simulink model "VSCHVDCunitblackstart"  (R2025b)
settings: Solver=VariableStepAuto  StartTime=0  StopTime=25  FixedStep=5e-5  RelTol=1e-3
PreLoadFcn:
  | HVDCParameters;
  | BlackStartMMCParameters;
undefined symbols (not defined in the file): DiscIntNeverNeededParam, FRated, frt, gGFM, grid, Lbase, Lr, Lt, lvrt, mGFM, mpptOmega, mpptWindSpeed, Nm, pmsm, PRated, Rc, rpir, Rr, Rt, time, Tpir, Ts, Vbase, Vdcs0, VRated, Vt2, windController, windTurbine, Zbase
libraries: fl_lib x47, ee_lib x41, nesl_utility x33, eeGeneralControl x13, eeTransforms x12, slpidlib x8, eeSinusoidalMeasurementV2 x4, simulink x2, eeSinusoidalMeasurement x1, eeStairGenerator x1
(part 2 of 5)

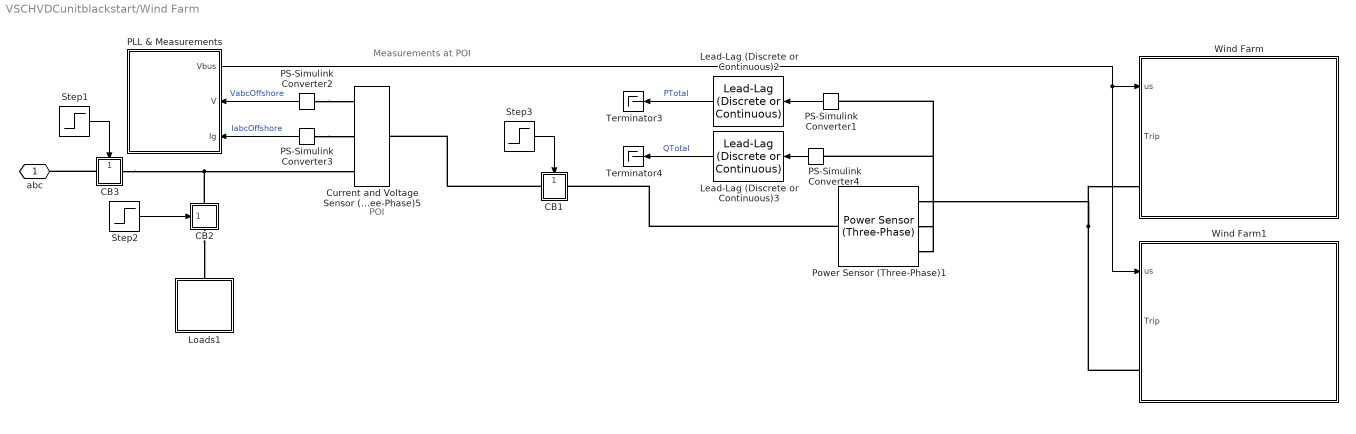
== system VSCHVDCunitblackstart/Wind Farm ==
  note: POI
  note: Measurements at POI
  CB1 : Subsystem
      settings: PortSchema="{\"entries\":[{\"content\":{\"sides\":[{\"content\":{\"connectorIds\":[\"LConn1\"]},\"type\":\"ConnectorPlacement.EquallySpacedRectSide\",\"uuid\":\"67c0f727-7c15-41c9-98df-b3c7d57498ed\"},{\"content\":{\"connectorIds\":[\"RConn1\"],\"side\":\"RIGHT\"},\"type\":\"ConnectorPlacement.EquallySpacedRectSide\",\"uuid\":\"7fc39429-ba61-416d-b42b-93e81eb2f426\"},{\"content\":{\"side\":\"TOP\"},\"type\":\"ConnectorPlacement.EquallySpacedRectSide\",\"uuid\":\"c6dd9263-b57a-4cff-a218-af99f2798f29\"},{\"content\":{\"connectorIds\":[\"In1\"],\"side\":\"BOTTOM\"},\"type\":\"ConnectorPlacement.EquallySpacedRectSide\",\"uuid\":\"e2a2ba44-d59d-4e27-adf1-3f94e828ca78\"}]},\"type\":\"ConnectorPlacement.EquallySpacedConnector\",\"uuid\":\"b349a99b-c902-4df9-9c99-34841afb28dd\"}],\"packageUris\":[\"http://schema.mathworks.com/mf0/Connector/R2020b\"],\"version\":\"1.0\"}"
  CB2 : Subsystem
      settings: PortSchema="{\"entries\":[{\"content\":{\"sides\":[{\"content\":{\"connectorIds\":[\"LConn1\"]},\"type\":\"ConnectorPlacement.EquallySpacedRectSide\",\"uuid\":\"67c0f727-7c15-41c9-98df-b3c7d57498ed\"},{\"content\":{\"connectorIds\":[\"RConn1\"],\"side\":\"RIGHT\"},\"type\":\"ConnectorPlacement.EquallySpacedRectSide\",\"uuid\":\"7fc39429-ba61-416d-b42b-93e81eb2f426\"},{\"content\":{\"side\":\"TOP\"},\"type\":\"ConnectorPlacement.EquallySpacedRectSide\",\"uuid\":\"c6dd9263-b57a-4cff-a218-af99f2798f29\"},{\"content\":{\"connectorIds\":[\"In1\"],\"side\":\"BOTTOM\"},\"type\":\"ConnectorPlacement.EquallySpacedRectSide\",\"uuid\":\"e2a2ba44-d59d-4e27-adf1-3f94e828ca78\"}]},\"type\":\"ConnectorPlacement.EquallySpacedConnector\",\"uuid\":\"b349a99b-c902-4df9-9c99-34841afb28dd\"}],\"packageUris\":[\"http://schema.mathworks.com/mf0/Connector/R2020b\"],\"version\":\"1.0\"}"
  CB3 : Subsystem
      settings: PortSchema="{\"entries\":[{\"content\":{\"sides\":[{\"content\":{\"connectorIds\":[\"LConn1\"]},\"type\":\"ConnectorPlacement.EquallySpacedRectSide\",\"uuid\":\"67c0f727-7c15-41c9-98df-b3c7d57498ed\"},{\"content\":{\"connectorIds\":[\"RConn1\"],\"side\":\"RIGHT\"},\"type\":\"ConnectorPlacement.EquallySpacedRectSide\",\"uuid\":\"7fc39429-ba61-416d-b42b-93e81eb2f426\"},{\"content\":{\"side\":\"TOP\"},\"type\":\"ConnectorPlacement.EquallySpacedRectSide\",\"uuid\":\"c6dd9263-b57a-4cff-a218-af99f2798f29\"},{\"content\":{\"connectorIds\":[\"In1\"],\"side\":\"BOTTOM\"},\"type\":\"ConnectorPlacement.EquallySpacedRectSide\",\"uuid\":\"e2a2ba44-d59d-4e27-adf1-3f94e828ca78\"}]},\"type\":\"ConnectorPlacement.EquallySpacedConnector\",\"uuid\":\"b349a99b-c902-4df9-9c99-34841afb28dd\"}],\"packageUris\":[\"http://schema.mathworks.com/mf0/Connector/R2020b\"],\"version\":\"1.0\"}"
  Current and Voltage Sensor (Three-Phase)5 : ee_lib/Sensors & Transducers/Current and Voltage Sensor (Three-Phase)  vMeasurementType=ee.enum.vmeasurement.lg  outputUnit=ee.enum.unit.pu  SRated=base.mVA A*V  VRated=base.kV V  I_specify=off  I_priority=None  I=[0, 0, 0] A  I_nominal_specify=off  I_nominal_value=1  I_nominal_unit=A  V_specify=off  V_priority=None  V=[0, 0, 0] V  V_nominal_specify=off  V_nominal_value=1  V_nominal_unit=V
      settings: InternalSimscapePortConfiguration="{\"Bottom\":[],\"Left\":[{\"id\":\"N1\",\"label\":\"~1\",\"type\":\"foundation.electrical.three_phase\"}],\"Right\":[{\"id\":\"V_output\",\"label\":\"V\",\"type\":\"output\"},{\"id\":\"I_output\",\"label\":\"I\",\"type\":\"output\"},{\"id\":\"N2\",\"label\":\"~2\",\"type\":\"foundation.electrical.three_phase\"}],\"Top\":[]}"
  Lead-Lag (Discrete or Continuous)2 : eeGeneralControl/Lead-Lag (Discrete or Continuous)  T1=0  T2=windController.tSensor  B=inf  A=-inf  init_option=Inherited from block input  x0=0  Ts=Ts
      settings: LibrarySourceBlock=|
      | ee_sl_lib/General Control/Lead-Lag
      | (Discrete or Continuous)
  Lead-Lag (Discrete or Continuous)3 : eeGeneralControl/Lead-Lag (Discrete or Continuous)  T1=0  T2=windController.tSensor  B=inf  A=-inf  init_option=Inherited from block input  x0=0  Ts=Ts
      settings: LibrarySourceBlock=|
      | ee_sl_lib/General Control/Lead-Lag
      | (Discrete or Continuous)
  Loads1 : Subsystem
      mask Display: image('Load_2.png');
  PLL & Measurements : Subsystem
      settings: PortSchema="{\"entries\":[{\"content\":{\"sides\":[{\"content\":{\"connectorIds\":[\"Out1\",\"In1\",\"In2\"]},\"type\":\"ConnectorPlacement.EquallySpacedRectSide\",\"uuid\":\"76485780-20fe-4fcf-8224-69648da6ed2a\"},{\"content\":{\"side\":\"RIGHT\"},\"type\":\"ConnectorPlacement.EquallySpacedRectSide\",\"uuid\":\"f19a6390-e634-42c7-8d46-4cd80cbab182\"},{\"content\":{\"side\":\"TOP\"},\"type\":\"ConnectorPlacement.EquallySpacedRectSide\",\"uuid\":\"87682f72-1844-428e-be70-ad7ca3191ee3\"}]},\"type\":\"ConnectorPlacement.EquallySpacedConnector\",\"uuid\":\"f2136b07-48ec-402b-adb3-18c0bac2157c\"}],\"packageUris\":[\"http://schema.mathworks.com/mf0/Connector/R2020b\"],\"version\":\"1.0\"}"
      mask Display: image('measurements.png'); % Use "Edit Image" on toolstrip to change.
  PS-Simulink Converter{1..4} (4 alike) : nesl_utility/PS-Simulink Converter  PhysicalDomain=network_engine_domain  SubClassName=ps_output  LeftPortType=input  RightPortType=output  PseudoPeriodic=off  Frequencies=[]  VectorFormat=inherit  Unit=inherit  AffineConversion=off
  Power Sensor (Three-Phase)1 : ee_lib/Sensors & Transducers/Power Sensor (Three-Phase)  load_type=ee.enum.passive.type_balanced.balanced  f0=60 Hz
      settings: InternalSimscapePortConfiguration="{\"Bottom\":[],\"Left\":[{\"id\":\"N1\",\"label\":\"~1\",\"type\":\"foundation.electrical.three_phase\"}],\"Right\":[{\"id\":\"N2\",\"label\":\"~2\",\"type\":\"foundation.electrical.three_phase\"}],\"Top\":[{\"id\":\"Pm\",\"label\":\"P\",\"type\":\"output\"},{\"id\":\"Qm\",\"label\":\"Q\",\"type\":\"output\"}]}"
  Step1 : Step  Time=9  Before=1  After=0  SampleTime=Ts
  Step2 : Step  Time=3  Before=1  After=0  SampleTime=Ts
  Step3 : Step  Time=2  Before=1  After=0  SampleTime=Ts
  Terminator3 : Terminator
  Terminator4 : Terminator
  Wind Farm : Subsystem
      settings: PortSchema="{\"entries\":[{\"content\":{\"sides\":[{\"content\":{\"connectorIds\":[\"In1\",\"Out1\",\"LConn1\"]},\"type\":\"ConnectorPlacement.EquallySpacedRectSide\",\"uuid\":\"1189e956-e6f0-4ada-905a-6b9abec668a8\"},{\"content\":{\"side\":\"RIGHT\"},\"type\":\"ConnectorPlacement.EquallySpacedRectSide\",\"uuid\":\"3ddb8f28-1c9c-423f-814f-a5e5ca919d79\"},{\"content\":{\"side\":\"TOP\"},\"type\":\"ConnectorPlacement.EquallySpacedRectSide\",\"uuid\":\"c360f229-efd7-488e-97f8-90fd9e6e05d4\"},{\"content\":{\"side\":\"BOTTOM\"},\"type\":\"ConnectorPlacement.EquallySpacedRectSide\",\"uuid\":\"99811ca4-1621-4e62-9767-ce3bd58f839c\"}]},\"type\":\"ConnectorPlacement.EquallySpacedConnector\",\"uuid\":\"16843f42-9f9b-4252-a0c2-a64badb15c83\"}],\"packageUris\":[\"http://schema.mathworks.com/mf0/Connector/R2020b\"],\"version\":\"1.0\"}"
      mask Display: image('WindFarmModel4_1.PNG');
  Wind Farm1 : Subsystem
      settings: PortSchema="{\"entries\":[{\"content\":{\"sides\":[{\"content\":{\"connectorIds\":[\"In1\",\"Out1\",\"LConn1\"]},\"type\":\"ConnectorPlacement.EquallySpacedRectSide\",\"uuid\":\"1189e956-e6f0-4ada-905a-6b9abec668a8\"},{\"content\":{\"side\":\"RIGHT\"},\"type\":\"ConnectorPlacement.EquallySpacedRectSide\",\"uuid\":\"3ddb8f28-1c9c-423f-814f-a5e5ca919d79\"},{\"content\":{\"side\":\"TOP\"},\"type\":\"ConnectorPlacement.EquallySpacedRectSide\",\"uuid\":\"c360f229-efd7-488e-97f8-90fd9e6e05d4\"},{\"content\":{\"side\":\"BOTTOM\"},\"type\":\"ConnectorPlacement.EquallySpacedRectSide\",\"uuid\":\"99811ca4-1621-4e62-9767-ce3bd58f839c\"}]},\"type\":\"ConnectorPlacement.EquallySpacedConnector\",\"uuid\":\"16843f42-9f9b-4252-a0c2-a64badb15c83\"}],\"packageUris\":[\"http://schema.mathworks.com/mf0/Connector/R2020b\"],\"version\":\"1.0\"}"
      mask Display: image('WindFarmModel4_1.PNG');
  abc : PMIOPort  Side=Right
  wires:
  PS-Simulink Converter2/1 -> PLL & Measurements/1(V)  "VabcOffshore"
  PS-Simulink Converter3/1 -> PLL & Measurements/2(Ig)  "IabcOffshore"
  Step3/1 -> CB1/1(input0)
  Step2/1 -> CB2/1(input0)
  PLL & Measurements/1(Vbus) -> Wind Farm1/1(us), Wind Farm/1(us)
  Step1/1 -> CB3/1(input0)
  Lead-Lag (Discrete or Continuous)2/1 -> Terminator3/1  "PTotal"
  PS-Simulink Converter1/1 -> Lead-Lag (Discrete or Continuous)2/1
  PS-Simulink Converter4/1 -> Lead-Lag (Discrete or Continuous)3/1
  Lead-Lag (Discrete or Continuous)3/1 -> Terminator4/1  "QTotal"
  connections:
  CB2/RConn1 -- CB3/RConn1 -- Current and Voltage Sensor (Three-Phase)5/RConn3
  CB2/LConn1 -- Loads1/RConn1
  CB1/LConn1 -- Current and Voltage Sensor (Three-Phase)5/LConn1
  PS-Simulink Converter2/LConn1 -- Current and Voltage Sensor (Three-Phase)5/RConn1
  PS-Simulink Converter3/LConn1 -- Current and Voltage Sensor (Three-Phase)5/RConn2
  Wind Farm1/LConn1 -- Power Sensor (Three-Phase)1/LConn1 -- Wind Farm/LConn1
  CB3/LConn1 -- abc/RConn1
  Power Sensor (Three-Phase)1/LConn3 -- PS-Simulink Converter4/LConn1
  Power Sensor (Three-Phase)1/LConn2 -- PS-Simulink Converter1/LConn1
  Power Sensor (Three-Phase)1/RConn1 -- CB1/RConn1

== system VSCHVDCunitblackstart/Cables/Idcnr ==
  Current Sensor : fl_lib/Electrical/Electrical Sensors/Current Sensor
  PS-Simulink Converter : nesl_utility/PS-Simulink Converter  PhysicalDomain=network_engine_domain  SubClassName=ps_output  LeftPortType=input  RightPortType=output  PseudoPeriodic=off  Frequencies=[]  VectorFormat=1-D array  Unit=A  AffineConversion=off
  + : PMIOPort  Side=Left
  - : PMIOPort  Port=2  Side=Right
  i : Outport
  wires:
  PS-Simulink Converter/1 -> i/1
  connections:
  -/RConn1 -- Current Sensor/RConn2
  Current Sensor/LConn1 -- +/RConn1
  PS-Simulink Converter/LConn1 -- Current Sensor/RConn1

== system VSCHVDCunitblackstart/Cables/Idcns ==
  Current Sensor : fl_lib/Electrical/Electrical Sensors/Current Sensor
  PS-Simulink Converter : nesl_utility/PS-Simulink Converter  PhysicalDomain=network_engine_domain  SubClassName=ps_output  LeftPortType=input  RightPortType=output  PseudoPeriodic=off  Frequencies=[]  VectorFormat=1-D array  Unit=A  AffineConversion=off
  + : PMIOPort  Side=Left
  - : PMIOPort  Port=2  Side=Right
  i : Outport
  wires:
  PS-Simulink Converter/1 -> i/1
  connections:
  PS-Simulink Converter/LConn1 -- Current Sensor/RConn1
  Current Sensor/LConn1 -- +/RConn1
  -/RConn1 -- Current Sensor/RConn2

== system VSCHVDCunitblackstart/Cables/Idcpr ==
  Current Sensor : fl_lib/Electrical/Electrical Sensors/Current Sensor
  PS-Simulink Converter : nesl_utility/PS-Simulink Converter  PhysicalDomain=network_engine_domain  SubClassName=ps_output  LeftPortType=input  RightPortType=output  PseudoPeriodic=off  Frequencies=[]  VectorFormat=1-D array  Unit=A  AffineConversion=off
  + : PMIOPort  Side=Left
  - : PMIOPort  Port=2  Side=Right
  i : Outport
  wires:
  PS-Simulink Converter/1 -> i/1
  connections:
  PS-Simulink Converter/LConn1 -- Current Sensor/RConn1
  Current Sensor/LConn1 -- +/RConn1
  -/RConn1 -- Current Sensor/RConn2

== system VSCHVDCunitblackstart/Cables/Idcps ==
  Current Sensor : fl_lib/Electrical/Electrical Sensors/Current Sensor
  PS-Simulink Converter : nesl_utility/PS-Simulink Converter  PhysicalDomain=network_engine_domain  SubClassName=ps_output  LeftPortType=input  RightPortType=output  PseudoPeriodic=off  Frequencies=[]  VectorFormat=1-D array  Unit=A  AffineConversion=off
  + : PMIOPort  Side=Left
  - : PMIOPort  Port=2  Side=Right
  i : Outport
  wires:
  PS-Simulink Converter/1 -> i/1
  connections:
  -/RConn1 -- Current Sensor/RConn2
  Current Sensor/LConn1 -- +/RConn1
  PS-Simulink Converter/LConn1 -- Current Sensor/RConn1

== system VSCHVDCunitblackstart/Cables/Vdcnr ==
  PS-Simulink Converter : nesl_utility/PS-Simulink Converter  PhysicalDomain=network_engine_domain  SubClassName=ps_output  LeftPortType=input  RightPortType=output  PseudoPeriodic=off  Frequencies=[]  VectorFormat=1-D array  Unit=V  AffineConversion=off
  Voltage Sensor : fl_lib/Electrical/Electrical Sensors/Voltage Sensor
  + : PMIOPort  Side=Left
  - : PMIOPort  Port=2  Side=Right
  v : Outport
  wires:
  PS-Simulink Converter/1 -> v/1
  connections:
  PS-Simulink Converter/LConn1 -- Voltage Sensor/RConn1
  Voltage Sensor/RConn2 -- -/RConn1
  Voltage Sensor/LConn1 -- +/RConn1

== system VSCHVDCunitblackstart/Cables/Vdcns ==
  PS-Simulink Converter : nesl_utility/PS-Simulink Converter  PhysicalDomain=network_engine_domain  SubClassName=ps_output  LeftPortType=input  RightPortType=output  PseudoPeriodic=off  Frequencies=[]  VectorFormat=1-D array  Unit=V  AffineConversion=off
  Voltage Sensor : fl_lib/Electrical/Electrical Sensors/Voltage Sensor
  + : PMIOPort  Side=Left
  - : PMIOPort  Port=2  Side=Right
  v : Outport
  wires:
  PS-Simulink Converter/1 -> v/1
  connections:
  Voltage Sensor/LConn1 -- +/RConn1
  Voltage Sensor/RConn2 -- -/RConn1
  PS-Simulink Converter/LConn1 -- Voltage Sensor/RConn1

== system VSCHVDCunitblackstart/Cables/Vdcpr ==
  PS-Simulink Converter : nesl_utility/PS-Simulink Converter  PhysicalDomain=network_engine_domain  SubClassName=ps_output  LeftPortType=input  RightPortType=output  PseudoPeriodic=off  Frequencies=[]  VectorFormat=1-D array  Unit=V  AffineConversion=off
  Voltage Sensor : fl_lib/Electrical/Electrical Sensors/Voltage Sensor
  + : PMIOPort  Side=Left
  - : PMIOPort  Port=2  Side=Right
  v : Outport
  wires:
  PS-Simulink Converter/1 -> v/1
  connections:
  Voltage Sensor/LConn1 -- +/RConn1
  Voltage Sensor/RConn2 -- -/RConn1
  PS-Simulink Converter/LConn1 -- Voltage Sensor/RConn1

== system VSCHVDCunitblackstart/Cables/Vdcps ==
  PS-Simulink Converter : nesl_utility/PS-Simulink Converter  PhysicalDomain=network_engine_domain  SubClassName=ps_output  LeftPortType=input  RightPortType=output  PseudoPeriodic=off  Frequencies=[]  VectorFormat=1-D array  Unit=V  AffineConversion=off
  Voltage Sensor : fl_lib/Electrical/Electrical Sensors/Voltage Sensor
  + : PMIOPort  Side=Left
  - : PMIOPort  Port=2  Side=Right
  v : Outport
  wires:
  PS-Simulink Converter/1 -> v/1
  connections:
  PS-Simulink Converter/LConn1 -- Voltage Sensor/RConn1
  Voltage Sensor/RConn2 -- -/RConn1
  Voltage Sensor/LConn1 -- +/RConn1

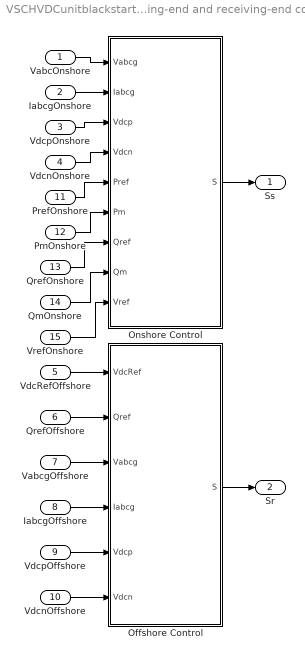
== system VSCHVDCunitblackstart/Control/Sending-end and receiving-end control ==
  VabcOnshore : Inport
  IabcgOnshore : Inport  Port=2
  VdcpOnshore : Inport  Port=3
  VdcnOnshore : Inport  Port=4
  VdcRefOffshore : Inport  Port=5
  QrefOffshore : Inport  Port=6
  VabcgOffshore : Inport  Port=7
  IabcgOffshore : Inport  Port=8
  VdcpOffshore : Inport  Port=9
  VdcnOffshore : Inport  Port=10
  PrefOnshore : Inport  Port=11
  PmOnshore : Inport  Port=12
  QrefOnshore : Inport  Port=13
  QmOnshore : Inport  Port=14
  VrefOnshore : Inport  Port=15
  Offshore Control : Subsystem  VariantControl=ControllerTimeMode
  Onshore Control : Subsystem  VariantControl=ControllerTimeMode
  Ss : Outport
  Sr : Outport  Port=2
  wires:
  QrefOffshore/1 -> Offshore Control/2(Qref)
  VabcgOffshore/1 -> Offshore Control/3(Vabcg)
  VdcnOffshore/1 -> Offshore Control/6(Vdcn)
  VdcpOffshore/1 -> Offshore Control/5(Vdcp)
  VdcnOnshore/1 -> Onshore Control/4(Vdcn)
  VdcRefOffshore/1 -> Offshore Control/1(VdcRef)
  Offshore Control/1(S) -> Sr/1
  IabcgOffshore/1 -> Offshore Control/4(Iabcg)
  IabcgOnshore/1 -> Onshore Control/2(Iabcg)
  VdcpOnshore/1 -> Onshore Control/3(Vdcp)
  VabcOnshore/1 -> Onshore Control/1(Vabcg)
  Onshore Control/1(S) -> Ss/1
  PrefOnshore/1 -> Onshore Control/5(Pref)
  PmOnshore/1 -> Onshore Control/6(Pm)
  QrefOnshore/1 -> Onshore Control/7(Qref)
  QmOnshore/1 -> Onshore Control/8(Qm)
  VrefOnshore/1 -> Onshore Control/9(Vref)

== system VSCHVDCunitblackstart/Offshore Station/Receiving-end vi ==
  Current and Voltage Sensor (Three-Phase) : ee_lib/Sensors & Transducers/Current and Voltage Sensor (Three-Phase)  vMeasurementType=ee.enum.vmeasurement.lg  outputUnit=ee.enum.unit.pu  SRated=PRated W  VRated=VgridRated V  I_specify=off  I_priority=None  I=[0, 0, 0] A  I_nominal_specify=off  I_nominal_value=1  I_nominal_unit=A  V_specify=off  V_priority=None  V=[0, 0, 0] V  V_nominal_specify=off  V_nominal_value=1  V_nominal_unit=V
      settings: InternalSimscapePortConfiguration="{\"Bottom\":[],\"Left\":[{\"id\":\"N1\",\"label\":\"~1\",\"type\":\"foundation.electrical.three_phase\"}],\"Right\":[{\"id\":\"V_output\",\"label\":\"V\",\"type\":\"output\"},{\"id\":\"I_output\",\"label\":\"I\",\"type\":\"output\"},{\"id\":\"N2\",\"label\":\"~2\",\"type\":\"foundation.electrical.three_phase\"}],\"Top\":[]}"
  PS-Simulink Converter : nesl_utility/PS-Simulink Converter  PhysicalDomain=network_engine_domain  SubClassName=ps_output  LeftPortType=input  RightPortType=output  PseudoPeriodic=off  Frequencies=[]  VectorFormat=1-D array  Unit=1  AffineConversion=off
  PS-Simulink Converter2 : nesl_utility/PS-Simulink Converter  PhysicalDomain=network_engine_domain  SubClassName=ps_output  LeftPortType=input  RightPortType=output  PseudoPeriodic=off  Frequencies=[]  VectorFormat=1-D array  Unit=1  AffineConversion=off
  ~1 : PMIOPort  Side=Left
  ~2 : PMIOPort  Port=2  Side=Right
  v : Outport
  i : Outport  Port=2
  wires:
  PS-Simulink Converter/1 -> i/1
  PS-Simulink Converter2/1 -> v/1
  connections:
  Current and Voltage Sensor (Three-Phase)/LConn1 -- ~1/RConn1
  Current and Voltage Sensor (Three-Phase)/RConn2 -- PS-Simulink Converter/LConn1
  PS-Simulink Converter2/LConn1 -- Current and Voltage Sensor (Three-Phase)/RConn1
  ~2/RConn1 -- Current and Voltage Sensor (Three-Phase)/RConn3

== system VSCHVDCunitblackstart/Onshore Grid/CB1 ==
  input0 : Inport
  Subsystem1 : Subsystem
      settings: PortSchema="{\"entries\":[{\"content\":{\"sides\":[{\"content\":{\"connectorIds\":[\"LConn1\",\"In1\"]},\"type\":\"ConnectorPlacement.EquallySpacedRectSide\",\"uuid\":\"4d523b2f-3490-490d-9193-0c3e52b1c3a1\"},{\"content\":{\"connectorIds\":[\"RConn1\"],\"side\":\"RIGHT\"},\"type\":\"ConnectorPlacement.EquallySpacedRectSide\",\"uuid\":\"1543a14a-65b5-4637-8d41-6da95a6ca307\"},{\"content\":{\"side\":\"TOP\"},\"type\":\"ConnectorPlacement.EquallySpacedRectSide\",\"uuid\":\"9fff8ee8-4727-466f-977a-681c4f14cc56\"}]},\"type\":\"ConnectorPlacement.EquallySpacedConnector\",\"uuid\":\"a46df766-bf17-4bd6-a8b3-579011040ee9\"}],\"packageUris\":[\"http://schema.mathworks.com/mf0/Connector/R2020b\"],\"version\":\"1.0\"}"
  Conn2 : PMIOPort  Side=Left
  Conn1 : PMIOPort  Port=2  Side=Right
  wires:
  input0/1 -> Subsystem1/1(input0)
  connections:
  Conn2/RConn1 -- Subsystem1/RConn1
  Subsystem1/LConn1 -- Conn1/RConn1

== system VSCHVDCunitblackstart/Onshore Grid/CB2 ==
  input0 : Inport
  Subsystem1 : Subsystem
      settings: PortSchema="{\"entries\":[{\"content\":{\"sides\":[{\"content\":{\"connectorIds\":[\"LConn1\",\"In1\"]},\"type\":\"ConnectorPlacement.EquallySpacedRectSide\",\"uuid\":\"4d523b2f-3490-490d-9193-0c3e52b1c3a1\"},{\"content\":{\"connectorIds\":[\"RConn1\"],\"side\":\"RIGHT\"},\"type\":\"ConnectorPlacement.EquallySpacedRectSide\",\"uuid\":\"1543a14a-65b5-4637-8d41-6da95a6ca307\"},{\"content\":{\"side\":\"TOP\"},\"type\":\"ConnectorPlacement.EquallySpacedRectSide\",\"uuid\":\"9fff8ee8-4727-466f-977a-681c4f14cc56\"}]},\"type\":\"ConnectorPlacement.EquallySpacedConnector\",\"uuid\":\"a46df766-bf17-4bd6-a8b3-579011040ee9\"}],\"packageUris\":[\"http://schema.mathworks.com/mf0/Connector/R2020b\"],\"version\":\"1.0\"}"
  Conn2 : PMIOPort  Side=Left
  Conn1 : PMIOPort  Port=2  Side=Right
  wires:
  input0/1 -> Subsystem1/1(input0)
  connections:
  Conn2/RConn1 -- Subsystem1/RConn1
  Subsystem1/LConn1 -- Conn1/RConn1

== system VSCHVDCunitblackstart/Onshore Grid/PLL & Measurements ==
  V : Inport
  Measurement2 : Subsystem
  PLL : Subsystem
  Out Bus Element2 : Outport  PortName=Vbus  Element=w
  Out Bus Element3 : Outport  PortName=Vbus  Element=Theta
  Out Bus Element4 : Outport  PortName=Vbus  Element=Vmag
  wires:
  V/1 -> Measurement2/1(u)
  PLL/2(freq) -> Out Bus Element2/1
  PLL/3(angle) -> Out Bus Element3/1
  Measurement2/1(Vg) -> PLL/1(abc)
  PLL/1(mag) -> Out Bus Element4/1  "Vmag"

== system VSCHVDCunitblackstart/Onshore Grid/Sending-end vi ==
  Current and Voltage Sensor (Three-Phase) : ee_lib/Sensors & Transducers/Current and Voltage Sensor (Three-Phase)  vMeasurementType=ee.enum.vmeasurement.lg  outputUnit=ee.enum.unit.pu  SRated=PRated W  VRated=VgridRated V  I_specify=off  I_priority=None  I=[0, 0, 0] A  I_nominal_specify=off  I_nominal_value=1  I_nominal_unit=A  V_specify=off  V_priority=None  V=[0, 0, 0] V  V_nominal_specify=off  V_nominal_value=1  V_nominal_unit=V
      settings: InternalSimscapePortConfiguration="{\"Bottom\":[],\"Left\":[{\"id\":\"N1\",\"label\":\"~1\",\"type\":\"foundation.electrical.three_phase\"}],\"Right\":[{\"id\":\"V_output\",\"label\":\"V\",\"type\":\"output\"},{\"id\":\"I_output\",\"label\":\"I\",\"type\":\"output\"},{\"id\":\"N2\",\"label\":\"~2\",\"type\":\"foundation.electrical.three_phase\"}],\"Top\":[]}"
  PS-Simulink Converter : nesl_utility/PS-Simulink Converter  PhysicalDomain=network_engine_domain  SubClassName=ps_output  LeftPortType=input  RightPortType=output  PseudoPeriodic=off  Frequencies=[]  VectorFormat=1-D array  Unit=1  AffineConversion=off
  PS-Simulink Converter2 : nesl_utility/PS-Simulink Converter  PhysicalDomain=network_engine_domain  SubClassName=ps_output  LeftPortType=input  RightPortType=output  PseudoPeriodic=off  Frequencies=[]  VectorFormat=1-D array  Unit=1  AffineConversion=off
  ~1 : PMIOPort  Side=Left
  ~2 : PMIOPort  Port=2  Side=Right
  v : Outport
  i : Outport  Port=2
  wires:
  PS-Simulink Converter2/1 -> v/1
  PS-Simulink Converter/1 -> i/1
  connections:
  PS-Simulink Converter2/LConn1 -- Current and Voltage Sensor (Three-Phase)/RConn1
  Current and Voltage Sensor (Three-Phase)/RConn2 -- PS-Simulink Converter/LConn1
  Current and Voltage Sensor (Three-Phase)/LConn1 -- ~1/RConn1
  ~2/RConn1 -- Current and Voltage Sensor (Three-Phase)/RConn3

== system VSCHVDCunitblackstart/PIR/Subsystem1 ==
  input0 : Inport
  Phase Splitter : ee_lib/Connectors & References/Phase Splitter
  Phase Splitter1 : ee_lib/Connectors & References/Phase Splitter
  Simulink-PS Converter : nesl_utility/Simulink-PS Converter  PhysicalDomain=network_engine_domain  SubClassName=ps_input  LeftPortType=input  RightPortType=output  PseudoPeriodic=off  Frequencies=[]  NoiseDistribution=none  NoiseParameters=[]  Unit=1  AffineConversion=off  FilteringAndDerivatives=provide  SimscapeFilterOrder=1  InputFilterTimeConstant=0.001  UdotUserProvided=0
  Variable Resistor : fl_lib/Electrical/Electrical Elements/Variable Resistor  Rmin=1e-4 Ohm  thermalEnable=false  thermal_mass=1 J/K  i_specify=off  i_priority=None  i=0 A  i_nominal_specify=off  i_nominal_value=1  i_nominal_unit=A  v_specify=off  v_priority=None  v=0 V  v_nominal_specify=off  v_nominal_value=1  v_nominal_unit=V  T_specify=off  T_priority=None  T=300 K  T_nominal_specify=off  T_nominal_value=1  T_nominal_unit=K
  Variable Resistor1 : fl_lib/Electrical/Electrical Elements/Variable Resistor  Rmin=1e-4 Ohm  thermalEnable=false  thermal_mass=1 J/K  i_specify=off  i_priority=None  i=0 A  i_nominal_specify=off  i_nominal_value=1  i_nominal_unit=A  v_specify=off  v_priority=None  v=0 V  v_nominal_specify=off  v_nominal_value=1  v_nominal_unit=V  T_specify=off  T_priority=None  T=300 K  T_nominal_specify=off  T_nominal_value=1  T_nominal_unit=K
  Variable Resistor2 : fl_lib/Electrical/Electrical Elements/Variable Resistor  Rmin=1e-4 Ohm  thermalEnable=false  thermal_mass=1 J/K  i_specify=off  i_priority=None  i=0 A  i_nominal_specify=off  i_nominal_value=1  i_nominal_unit=A  v_specify=off  v_priority=None  v=0 V  v_nominal_specify=off  v_nominal_value=1  v_nominal_unit=V  T_specify=off  T_priority=None  T=300 K  T_nominal_specify=off  T_nominal_value=1  T_nominal_unit=K
  Conn1 : PMIOPort  Side=Left
  Conn2 : PMIOPort  Port=2  Side=Right
  wires:
  input0/1 -> Simulink-PS Converter/1
  connections:
  Simulink-PS Converter/RConn1 -- Variable Resistor2/LConn1 -- Variable Resistor1/LConn1 -- Variable Resistor/LConn1
  Phase Splitter/LConn1 -- Conn2/RConn1
  Phase Splitter/RConn1 -- Variable Resistor/LConn2
  Phase Splitter/RConn2 -- Variable Resistor1/LConn2
  Phase Splitter/RConn3 -- Variable Resistor2/LConn2
  Phase Splitter1/LConn1 -- Conn1/RConn1
  Variable Resistor/RConn1 -- Phase Splitter1/RConn1
  Phase Splitter1/RConn2 -- Variable Resistor1/RConn1
  Variable Resistor2/RConn1 -- Phase Splitter1/RConn3

== system VSCHVDCunitblackstart/Wind Farm/CB1 ==
  input0 : Inport
  Subsystem1 : Subsystem
      settings: PortSchema="{\"entries\":[{\"content\":{\"sides\":[{\"content\":{\"connectorIds\":[\"LConn1\",\"In1\"]},\"type\":\"ConnectorPlacement.EquallySpacedRectSide\",\"uuid\":\"4d523b2f-3490-490d-9193-0c3e52b1c3a1\"},{\"content\":{\"connectorIds\":[\"RConn1\"],\"side\":\"RIGHT\"},\"type\":\"ConnectorPlacement.EquallySpacedRectSide\",\"uuid\":\"1543a14a-65b5-4637-8d41-6da95a6ca307\"},{\"content\":{\"side\":\"TOP\"},\"type\":\"ConnectorPlacement.EquallySpacedRectSide\",\"uuid\":\"9fff8ee8-4727-466f-977a-681c4f14cc56\"}]},\"type\":\"ConnectorPlacement.EquallySpacedConnector\",\"uuid\":\"a46df766-bf17-4bd6-a8b3-579011040ee9\"}],\"packageUris\":[\"http://schema.mathworks.com/mf0/Connector/R2020b\"],\"version\":\"1.0\"}"
  Conn2 : PMIOPort  Side=Left
  Conn1 : PMIOPort  Port=2  Side=Right
  wires:
  input0/1 -> Subsystem1/1(input0)
  connections:
  Conn2/RConn1 -- Subsystem1/RConn1
  Subsystem1/LConn1 -- Conn1/RConn1

== system VSCHVDCunitblackstart/Wind Farm/CB2 ==
  input0 : Inport
  Subsystem1 : Subsystem
      settings: PortSchema="{\"entries\":[{\"content\":{\"sides\":[{\"content\":{\"connectorIds\":[\"LConn1\",\"In1\"]},\"type\":\"ConnectorPlacement.EquallySpacedRectSide\",\"uuid\":\"4d523b2f-3490-490d-9193-0c3e52b1c3a1\"},{\"content\":{\"connectorIds\":[\"RConn1\"],\"side\":\"RIGHT\"},\"type\":\"ConnectorPlacement.EquallySpacedRectSide\",\"uuid\":\"1543a14a-65b5-4637-8d41-6da95a6ca307\"},{\"content\":{\"side\":\"TOP\"},\"type\":\"ConnectorPlacement.EquallySpacedRectSide\",\"uuid\":\"9fff8ee8-4727-466f-977a-681c4f14cc56\"}]},\"type\":\"ConnectorPlacement.EquallySpacedConnector\",\"uuid\":\"a46df766-bf17-4bd6-a8b3-579011040ee9\"}],\"packageUris\":[\"http://schema.mathworks.com/mf0/Connector/R2020b\"],\"version\":\"1.0\"}"
  Conn2 : PMIOPort  Side=Left
  Conn1 : PMIOPort  Port=2  Side=Right
  wires:
  input0/1 -> Subsystem1/1(input0)
  connections:
  Conn2/RConn1 -- Subsystem1/RConn1
  Subsystem1/LConn1 -- Conn1/RConn1

== system VSCHVDCunitblackstart/Wind Farm/CB3 ==
  input0 : Inport
  Subsystem1 : Subsystem
      settings: PortSchema="{\"entries\":[{\"content\":{\"sides\":[{\"content\":{\"connectorIds\":[\"LConn1\",\"In1\"]},\"type\":\"ConnectorPlacement.EquallySpacedRectSide\",\"uuid\":\"4d523b2f-3490-490d-9193-0c3e52b1c3a1\"},{\"content\":{\"connectorIds\":[\"RConn1\"],\"side\":\"RIGHT\"},\"type\":\"ConnectorPlacement.EquallySpacedRectSide\",\"uuid\":\"1543a14a-65b5-4637-8d41-6da95a6ca307\"},{\"content\":{\"side\":\"TOP\"},\"type\":\"ConnectorPlacement.EquallySpacedRectSide\",\"uuid\":\"9fff8ee8-4727-466f-977a-681c4f14cc56\"}]},\"type\":\"ConnectorPlacement.EquallySpacedConnector\",\"uuid\":\"a46df766-bf17-4bd6-a8b3-579011040ee9\"}],\"packageUris\":[\"http://schema.mathworks.com/mf0/Connector/R2020b\"],\"version\":\"1.0\"}"
  abc : PMIOPort  Side=Left
  Conn1 : PMIOPort  Port=2  Side=Right
  wires:
  input0/1 -> Subsystem1/1(input0)
  connections:
  abc/RConn1 -- Subsystem1/RConn1
  Subsystem1/LConn1 -- Conn1/RConn1

== system VSCHVDCunitblackstart/Wind Farm/Loads1 ==
  note: Load
  Electrical Reference4 : fl_lib/Electrical/Electrical Elements/Electrical Reference
  Wye-Connected Load : ee_lib/Passive/RLC Assemblies/Wye-Connected Load  port_option=ee.enum.threePhasePort.composite  parameterization=ee.enum.rlc.parameterization.ratedpower  component_structure=ee.enum.rlc.structure.R  component_structure_PQ=ee.enum.rlc.structure.R  R=1 Ohm  L=1e-3 H  C=1e-6 F  VRated=windTransformer.lv V  FRated=60 Hz  P=1e4 W  Qpos=1e2 A*V  Qneg=-1e2 A*V  R_parasitic=0 Ohm  G_parasitic=0 1/Ohm  R_parasitic_PQ=0 Ohm  G_parasitic_PQ=0 1/Ohm  Vmag0=24e3 V  Vang0=0 deg  Freq0=60 Hz  IL_specify=off  IL_priority=High  IL=[0, 0, 0] A  IL_nominal_specify=off  IL_nominal_value=1  IL_nominal_unit=A  VC_specify=off  VC_priority=High  VC=[0, 0, 0] V  VC_nominal_specify=off  VC_nominal_value=1  VC_nominal_unit=V
  Conn1 : PMIOPort  Side=Right
  connections:
  Electrical Reference4/LConn1 -- Wye-Connected Load/RConn1
  Wye-Connected Load/LConn1 -- Conn1/RConn1

== system VSCHVDCunitblackstart/Wind Farm/PLL & Measurements ==
  V : Inport
  Ig : Inport  Port=2
  Measurement1 : Subsystem
  Measurement2 : Subsystem
  PLL : Subsystem
  Out Bus Element : Outport  PortName=Vbus  Element=Vq
  Out Bus Element1 : Outport  PortName=Vbus  Element=Vd
  Out Bus Element2 : Outport  PortName=Vbus  Element=w
  Out Bus Element3 : Outport  PortName=Vbus  Element=Theta
  Out Bus Element4 : Outport  PortName=Vbus  Element=Vmag
  Out Bus Element5 : Outport  PortName=Vbus  Element=Id
  Out Bus Element6 : Outport  PortName=Vbus  Element=Iq
  wires:
  V/1 -> Measurement2/1(u)
  PLL/2(freq) -> Out Bus Element2/1
  PLL/5(Vq) -> Out Bus Element/1  "Vq"
  PLL/3(angle) -> Out Bus Element3/1
  PLL/4(Vd) -> Out Bus Element1/1
  Measurement2/1(Vg) -> PLL/1(abc)
  PLL/1(mag) -> Out Bus Element4/1  "Vmag"
  Measurement1/1(Ig) -> PLL/2(Ig)
  Ig/1 -> Measurement1/1(u)
  PLL/7(Iq) -> Out Bus Element6/1  "Iq"
  PLL/6(Id) -> Out Bus Element5/1  "Id"

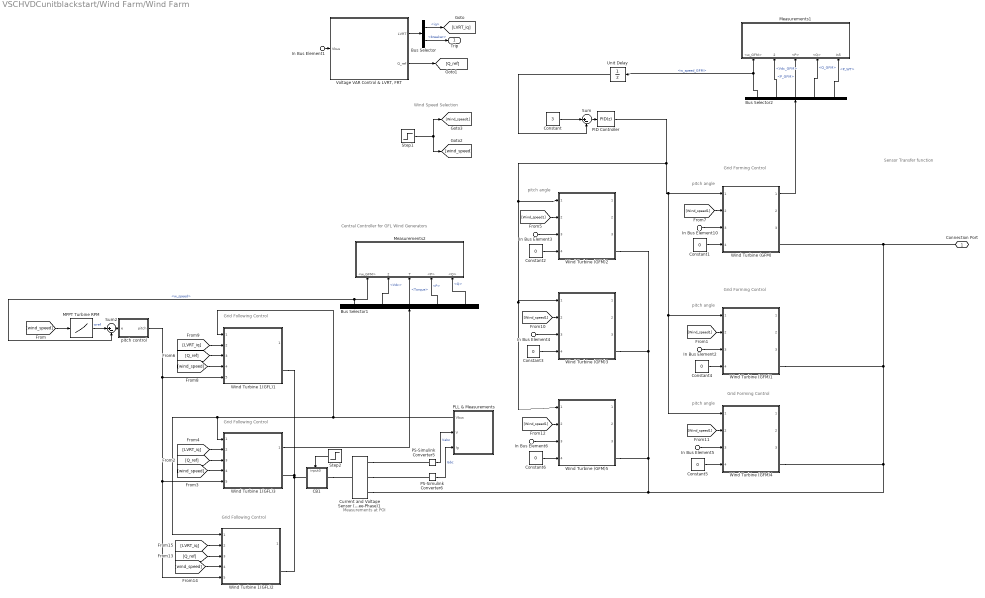
== system VSCHVDCunitblackstart/Wind Farm/Wind Farm ==
  note: Central Controller for GFL Wind Generators
  note: Wind Speed Selection
  note: Sensor Transfer function
  note: pitch angle
  note: Grid Forming Control
  note: Grid Forming Control
  note: pitch angle
  note: Grid Forming Control
  note: Measurements at POI
  note: pitch angle
  note: pitch angle
  note: Grid Following Control
  note: Grid Following Control
  note: Grid Following Control
  In Bus Element{1..6,10} (7 alike) : Inport  PortName=us
  Bus Selector : BusSelector  OutputSignals=iq,breaker
  Bus Selector1 : BusSelector  OutputSignals=w_speed,Vdc,Torque,P,Q
  Bus Selector2 : BusSelector  OutputSignals=w_speed_GFM,Vdc_GFM,P_GFM,Q_GFM,P_WT
  CB1 : Subsystem
      settings: PortSchema="{\"entries\":[{\"content\":{\"sides\":[{\"content\":{\"connectorIds\":[\"LConn1\"]},\"type\":\"ConnectorPlacement.EquallySpacedRectSide\",\"uuid\":\"67c0f727-7c15-41c9-98df-b3c7d57498ed\"},{\"content\":{\"connectorIds\":[\"RConn1\"],\"side\":\"RIGHT\"},\"type\":\"ConnectorPlacement.EquallySpacedRectSide\",\"uuid\":\"7fc39429-ba61-416d-b42b-93e81eb2f426\"},{\"content\":{\"side\":\"TOP\"},\"type\":\"ConnectorPlacement.EquallySpacedRectSide\",\"uuid\":\"c6dd9263-b57a-4cff-a218-af99f2798f29\"},{\"content\":{\"connectorIds\":[\"In1\"],\"side\":\"BOTTOM\"},\"type\":\"ConnectorPlacement.EquallySpacedRectSide\",\"uuid\":\"e2a2ba44-d59d-4e27-adf1-3f94e828ca78\"}]},\"type\":\"ConnectorPlacement.EquallySpacedConnector\",\"uuid\":\"b349a99b-c902-4df9-9c99-34841afb28dd\"}],\"packageUris\":[\"http://schema.mathworks.com/mf0/Connector/R2020b\"],\"version\":\"1.0\"}"
  Constant : Constant  Value=3
  Constant{1..6} (6 alike) : Constant  Value=0
  Current and Voltage Sensor (Three-Phase)1 : ee_lib/Sensors & Transducers/Current and Voltage Sensor (Three-Phase)  vMeasurementType=ee.enum.vmeasurement.lg  outputUnit=ee.enum.unit.pu  SRated=base.mVA A*V  VRated=base.kV V  I_specify=off  I_priority=None  I=[0, 0, 0] A  I_nominal_specify=off  I_nominal_value=1  I_nominal_unit=A  V_specify=off  V_priority=None  V=[0, 0, 0] V  V_nominal_specify=off  V_nominal_value=1  V_nominal_unit=V
      settings: InternalSimscapePortConfiguration="{\"Bottom\":[],\"Left\":[{\"id\":\"N1\",\"label\":\"~1\",\"type\":\"foundation.electrical.three_phase\"}],\"Right\":[{\"id\":\"V_output\",\"label\":\"V\",\"type\":\"output\"},{\"id\":\"I_output\",\"label\":\"I\",\"type\":\"output\"},{\"id\":\"N2\",\"label\":\"~2\",\"type\":\"foundation.electrical.three_phase\"}],\"Top\":[]}"
  MPPT Turbine RPM : Lookup_n-D  NumberOfTableDimensions=1  BreakpointsForDimension1=mpptWindSpeed  Table=mpptOmega  InternalRulePriority=Speed  RndMeth=Simplest
  Measurements1 : Subsystem
  Measurements2 : Subsystem
  PID Controller : slpidlib/PID Controller  Controller=PID  Form=Parallel  TimeDomain=Discrete-time  UseExternalTs=off  SampleTime=-1  IntegratorMethod=Forward Euler  FilterMethod=Forward Euler  ControllerParametersSource=internal  P=-0.5  I=-1  UseKiTs=off  D=0  UseExternalDerivativeSource=off  N=100  UseFilter=on  TunerSelectOption=Transfer Function Based (PID Tuner App)  InitialConditionSource=internal  InitialConditionForIntegrator=0  InitialConditionForFilter=0  DifferentiatorICPrevScaledInput=0  ExternalReset=none  TrackingMode=off  Kt=1  LimitOutput=off  SatLimitsSource=internal  UpperSaturationLimit=20  LowerSaturationLimit=-20  LinearizeAsGain=on  AntiWindupMode=back-calculation  Kb=1  LimitIntegrator=off  UpperIntegratorSaturationLimit=inf  LowerIntegratorSaturationLimit=-inf  POutMin=[]  POutMax=[]  IOutMin=[]  IOutMax=[]  DOutMin=[]  DOutMax=[]  NOutMin=[]  NOutMax=[]  SumOutMin=[]  SumOutMax=[]  SaturationOutMin=[]  SaturationOutMax=[]  PParamMin=[]  PParamMax=[]  IParamMin=[]  IParamMax=[]  DParamMin=[]  DParamMax=[]  NParamMin=[]  NParamMax=[]  KbParamMin=[]  KbParamMax=[]  KtParamMin=[]  KtParamMax=[]  KbOutMin=[]  KbOutMax=[]  KtOutMin=[]  KtOutMax=[]  IntegratorOutMin=[]  IntegratorOutMax=[]  FilterOutMin=[]  FilterOutMax=[]  SumI1OutMin=[]  SumI1OutMax=[]  SumI2OutMin=[]  SumI2OutMax=[]  SumI3OutMin=[]  SumI3OutMax=[]  SumI4OutMin=[]  SumI4OutMax=[]  SumDOutMin=[]  SumDOutMax=[]  DifferentiatorOutMin=[]  DifferentiatorOutMax=[]  FilterDiffOutCoefMin=[]  FilterDiffOutCoefMax=[]  ReciprocalOutMin=[]  ReciprocalOutMax=[]  SumDenOutMin=[]  SumDenOutMax=[]  SumNumOutMin=[]  SumNumOutMax=[]  DivideOutMin=[]  DivideOutMax=[]  UdiffTsProdOutMin=[]  UdiffTsProdOutMax=[]  NTsProdOutMin=[]  NTsProdOutMax=[]  UintegralTsProdOutMin=[]  UintegralTsProdOutMax=[]  UngainTsProdOutMin=[]  UngainTsProdOutMax=[]  ClampingZeroOutDataTypeStr=Inherit: Inherit via back propagation  ClampingZeroOutMin=[]  ClampingZeroOutMax=[]  FilterDenConstantOutDataTypeStr=Inherit: Inherit via back propagation  FilterDenConstantOutMin=[]  FilterDenConstantOutMax=[]  PCopyOutDataTypeStr=Inherit: Inherit via back propagation  PCopyOutMin=[]  PCopyOutMax=[]  NCopyOutDataTypeStr=Inherit: Inherit via back propagation  NCopyOutMin=[]  NCopyOutMax=[]  IntegratorContinuousStateAttributes=''  IntegratorStateMustResolveToSignalObject=off  IntegratorRTWStateStorageClass=Auto  FilterContinuousStateAttributes=''  FilterStateMustResolveToSignalObject=off  FilterRTWStateStorageClass=Auto  ParallelPVariant=InternalParameters  IdealPVariant=Disabled  IVariant=InternalParameters  DVariant=InternalParameters  IntegratorVariant=Discrete  SatVariant=Disabled  AWVariant=Passthrough  PCopyVariant=Disabled  TRVariant=Disabled  FdbkBlocksVariant=Forward  IdealPFdbkVariant=Disabled  SatFdbkVariant=Disabled  DerivativeFilterVariant=ForwardEulerFilter  NVariant=InternalParameters  NCopyVariant=Disabled  FilterICVariant=InternalICsFilter  IntegratorICVariant=InternalICs  ExternalResetVariant=Disabled  TRSumVariant=Passthrough  SumFdbkVariant=Disabled  SumVariant=Sum_PID  TsampFilterVariant=InternalTs  TsampNgainVariant=Passthrough  TsampIntegralVariant=Disabled_SignalSpec  ExternalSaturationOutDataTypeStr=Inherit: Same as second input  DerivativeSourceVariant=ErrorSignal  PreIntVariant=InternalPreInt
  PLL & Measurements : Subsystem
      settings: PortSchema="{\"entries\":[{\"content\":{\"sides\":[{\"content\":{\"connectorIds\":[\"Out1\",\"In1\",\"In2\"]},\"type\":\"ConnectorPlacement.EquallySpacedRectSide\",\"uuid\":\"76485780-20fe-4fcf-8224-69648da6ed2a\"},{\"content\":{\"side\":\"RIGHT\"},\"type\":\"ConnectorPlacement.EquallySpacedRectSide\",\"uuid\":\"f19a6390-e634-42c7-8d46-4cd80cbab182\"},{\"content\":{\"side\":\"TOP\"},\"type\":\"ConnectorPlacement.EquallySpacedRectSide\",\"uuid\":\"87682f72-1844-428e-be70-ad7ca3191ee3\"}]},\"type\":\"ConnectorPlacement.EquallySpacedConnector\",\"uuid\":\"f2136b07-48ec-402b-adb3-18c0bac2157c\"}],\"packageUris\":[\"http://schema.mathworks.com/mf0/Connector/R2020b\"],\"version\":\"1.0\"}"
      mask Display: image('measurements.png'); % Use "Edit Image" on toolstrip to change.
  PS-Simulink Converter5 : nesl_utility/PS-Simulink Converter  PhysicalDomain=network_engine_domain  SubClassName=ps_output  LeftPortType=input  RightPortType=output  PseudoPeriodic=off  Frequencies=[]  VectorFormat=inherit  Unit=inherit  AffineConversion=off
  PS-Simulink Converter6 : nesl_utility/PS-Simulink Converter  PhysicalDomain=network_engine_domain  SubClassName=ps_output  LeftPortType=input  RightPortType=output  PseudoPeriodic=off  Frequencies=[]  VectorFormat=inherit  Unit=inherit  AffineConversion=off
  Step1 : Step  Time=time.wind  Before=11  After=11  SampleTime=5e-5  ZeroCross=off
  Step2 : Step  Time=6  Before=1  After=0  SampleTime=Ts
  Sum : Sum  Inputs=|+-
  Sum2 : Sum  Inputs=|+-
  Unit Delay : UnitDelay  SampleTime=-1  HasFrameUpgradeWarning=on
  "Voltage VAR Control & LVRT, FRT" : Subsystem
      mask Display: image('LVRT_4.png');
  Wind Turbine (GFM){,1..5} (6 alike) : Subsystem  ReferencedSubsystem=gfmWind  Control=VSM Using Turbine Inertia  V_ref=gGFM.vref  Q_ref=gGFM.qref  Kq=gGFM.kq  Kt=gGFM.kt  KqI=mGFM.kq  Kp=mGFM.kp*10  Kd=gGFM.kd  Kj=gGFM.kj  H=mGFM.h  D=mGFM.d  Vd_ref=mGFM.Vd  frequency1=gGFM.fref  frequency=mGFM.fref  Spref=Curtailed Power Operation  tstart=0  Vslope=1  Pstart=1  Pslope=1  x_vir=mGFM.x_vir  x_vir1=gGFM.r_vir  r_vir1=gGFM.x_vir  Imax1=gGFM.Imax  Imax=mGFM.Imax  r_vir=mGFM.r_vir  Kpq_mpp=pmsm.lq*pmsm.alpha  Kpd_mpp=pmsm.ld*pmsm.alpha  Kiq_mpp=pmsm.rs*pmsm.alpha  Kid_mpp=pmsm.rs*pmsm.alpha  Kpq=pmsm.lq*pmsm.alpha  Kpd=pmsm.ld*pmsm.alpha  Kiq=pmsm.rs*pmsm.alpha  Kid=pmsm.rs*pmsm.alpha  Kp_dc_sm=mGFM.kpdc  Ki_dc_sm=mGFM.kidc  wt1=0.01  rt1=0.01  pitch1=windTurbine.pitch  cp1=windTurbine.cp  airDensity1=windTurbine.airDensity  TSR1=windTurbine.TSR  Radius1=windTurbine.turbineRadius  wt=0.01  rt=0.01  pitch=windTurbine.pitch  cp=windTurbine.cp  airDensity=windTurbine.airDensity  Radius=windTurbine.turbineRadius  TSR=windTurbine.TSR  Inertia1=windTurbine.inertia  Inertia=windTurbine.inertia  psim1=pmsm.psim  p1=pmsm.p  Rs1=pmsm.rs  Lq1=pmsm.lq  Ld1=pmsm.ld  Ld=pmsm.ld  Lq=pmsm.lq  Rs=pmsm.rs  p=pmsm.p  psim=pmsm.psim
  Wind Turbine 1(GFL)1 : Subsystem  ReferencedSubsystem=WindGFLMpp  p=pmsm.p  psim=pmsm.psim  Rs=pmsm.rs  Ld=pmsm.ld  Lq=pmsm.lq  Kdip_sm=pmsm.ld*pmsm.alpha  Kdii_sm=pmsm.rs*pmsm.alpha  Kqip_sm=pmsm.lq*pmsm.alpha  Kqii_sm=pmsm.rs*pmsm.alpha  airDensity=windTurbine.airDensity  turbineRadius=windTurbine.turbineRadius  pitch=windTurbine.pitch  TSR=windTurbine.TSR  cp=windTurbine.cp  wt=0.01  rt=0.01  Inertia=windTurbine.inertia/100  Kp_dc=windController.kpv  Ki_dc=windController.kiv  Kdpi_g=windController.kpic  Kdii_g=windController.kiic  Kqpi_g=windController.kpic  Kqii_g=windController.kiic  blk=Enabled  slop=0.8  tst=6
  Wind Turbine 1(GFL)2 : Subsystem  ReferencedSubsystem=WindGFLMpp  p=pmsm.p  psim=pmsm.psim  Rs=pmsm.rs  Ld=pmsm.ld  Lq=pmsm.lq  Kdip_sm=pmsm.ld*pmsm.alpha  Kdii_sm=pmsm.rs*pmsm.alpha  Kqip_sm=pmsm.lq*pmsm.alpha  Kqii_sm=pmsm.rs*pmsm.alpha  airDensity=windTurbine.airDensity  turbineRadius=windTurbine.turbineRadius  pitch=windTurbine.pitch  TSR=windTurbine.TSR  cp=windTurbine.cp  wt=0.01  rt=0.01  Inertia=windTurbine.inertia/100  Kp_dc=windController.kpv  Ki_dc=windController.kiv  Kdpi_g=windController.kpic  Kdii_g=windController.kiic  Kqpi_g=windController.kpic  Kqii_g=windController.kiic  blk=Enabled  slop=0.8  tst=6
  Wind Turbine 1(GFL)3 : Subsystem  ReferencedSubsystem=WindGFLMpp  p=pmsm.p  psim=pmsm.psim  Rs=pmsm.rs  Ld=pmsm.ld  Lq=pmsm.lq  Kdip_sm=pmsm.ld*pmsm.alpha  Kdii_sm=pmsm.rs*pmsm.alpha  Kqip_sm=pmsm.lq*pmsm.alpha  Kqii_sm=pmsm.rs*pmsm.alpha  airDensity=windTurbine.airDensity  turbineRadius=windTurbine.turbineRadius  pitch=windTurbine.pitch  TSR=windTurbine.TSR  cp=windTurbine.cp  wt=0.01  rt=0.01  Inertia=windTurbine.inertia/100  Kp_dc=windController.kpv  Ki_dc=windController.kiv  Kdpi_g=windController.kpic  Kdii_g=windController.kiic  Kqpi_g=windController.kpic  Kqii_g=windController.kiic  blk=Enabled  slop=0.8  tst=6
  pitch control : Subsystem
      mask Display: disp('Pitch Control')
  Connection Port : PMIOPort  Side=Left
  Trip : Outport
  wires:
  "Voltage VAR Control & LVRT, FRT"/1(LVRT) -> Bus Selector/1
  In Bus Element1/1 -> "Voltage VAR Control & LVRT, FRT"/1(Vbus)
  Bus Selector/2 -> Trip/1  "<breaker>"
  "Voltage VAR Control & LVRT, FRT"/2(Q_ref) -> [Q_ref]
  Bus Selector/1 -> [LVRT_iq]  "<iq>"
  Bus Selector2/4 -> Measurements1/4(<Q>)  "<Q_GFM>"
  Bus Selector2/3 -> Measurements1/3(<P>)  "<P_GFM>"
  Bus Selector2/1 -> Measurements1/1(<w_GFM>), Unit Delay/1  "<w_speed_GFM>"
  Bus Selector2/2 -> Measurements1/2(<Vdc_GFM>)  "<Vdc_GFM>"
  Wind Turbine (GFM)/1 -> Bus Selector2/1
  Step1/1 -> [Wind_speed1], [wind_speed]
  [Wind_speed1] -> Wind Turbine (GFM)/2
  In Bus Element10/1 -> Wind Turbine (GFM)/3
  Bus Selector2/5 -> Measurements1/5(In5)  "<P_WT>"
  Unit Delay/1 -> Sum/2
  Sum/1 -> PID Controller/1
  Constant/1 -> Sum/1
  [Wind_speed1] -> Wind Turbine (GFM)1/2
  In Bus Element2/1 -> Wind Turbine (GFM)1/3
  [LVRT_iq] -> Wind Turbine 1(GFL)3/2
  [Q_ref] -> Wind Turbine 1(GFL)3/3
  [wind_speed] -> Wind Turbine 1(GFL)3/4
  Bus Selector1/2 -> Measurements2/2(<Vdc_GFM>)  "<Vdc>"
  Bus Selector1/4 -> Measurements2/4(<P>)  "<P>"
  Bus Selector1/5 -> Measurements2/5(<Q>)  "<Q>"
  Bus Selector1/3 -> Measurements2/3(T)  "<Torque>"
  Wind Turbine 1(GFL)3/1 -> Bus Selector1/1
  [wind_speed] -> MPPT Turbine RPM/1
  MPPT Turbine RPM/1 -> Sum2/1  "wref"
  Bus Selector1/1 -> Measurements2/1(<w_GFM>), Sum2/2  "<w_speed>"
  Sum2/1 -> pitch control/1(e)
  PS-Simulink Converter5/1 -> PLL & Measurements/1(V)  "Vabc"
  PS-Simulink Converter6/1 -> PLL & Measurements/2(Ig)  "Iabc"
  Step2/1 -> CB1/1(input0)
  In Bus Element3/1 -> Wind Turbine (GFM)2/3
  [Wind_speed1] -> Wind Turbine (GFM)2/2
  [Q_ref] -> Wind Turbine 1(GFL)1/3
  pitch control/1(pitch) -> Wind Turbine 1(GFL)2/5, Wind Turbine 1(GFL)3/5, Wind Turbine 1(GFL)1/5
  [LVRT_iq] -> Wind Turbine 1(GFL)1/2
  [wind_speed] -> Wind Turbine 1(GFL)1/4
  [Wind_speed1] -> Wind Turbine (GFM)3/2
  In Bus Element4/1 -> Wind Turbine (GFM)3/3
  [Wind_speed1] -> Wind Turbine (GFM)4/2
  PID Controller/1 -> Wind Turbine (GFM)4/1, Wind Turbine (GFM)1/1, Wind Turbine (GFM)/1, Wind Turbine (GFM)5/1, Wind Turbine (GFM)3/1, Wind Turbine (GFM)2/1
  In Bus Element6/1 -> Wind Turbine (GFM)5/3
  [Wind_speed1] -> Wind Turbine (GFM)5/2
  In Bus Element5/1 -> Wind Turbine (GFM)4/3
  [LVRT_iq] -> Wind Turbine 1(GFL)2/2
  [Q_ref] -> Wind Turbine 1(GFL)2/3
  PLL & Measurements/1(Vbus) -> Wind Turbine 1(GFL)1/1, Wind Turbine 1(GFL)3/1, Wind Turbine 1(GFL)2/1
  [wind_speed] -> Wind Turbine 1(GFL)2/4
  Constant1/1 -> Wind Turbine (GFM)/4
  Constant2/1 -> Wind Turbine (GFM)2/4
  Constant3/1 -> Wind Turbine (GFM)3/4
  Constant4/1 -> Wind Turbine (GFM)1/4
  Constant5/1 -> Wind Turbine (GFM)4/4
  Constant6/1 -> Wind Turbine (GFM)5/4
  connections:
  Wind Turbine (GFM)1/RConn1 -- Wind Turbine (GFM)2/RConn1 -- Wind Turbine (GFM)3/RConn1 -- Wind Turbine (GFM)5/RConn1 -- Current and Voltage Sensor (Three-Phase)1/RConn3 -- Wind Turbine (GFM)4/RConn1 -- Connection Port/RConn1 -- Wind Turbine (GFM)/RConn1
  Current and Voltage Sensor (Three-Phase)1/RConn1 -- PS-Simulink Converter5/LConn1
  Current and Voltage Sensor (Three-Phase)1/RConn2 -- PS-Simulink Converter6/LConn1
  Wind Turbine 1(GFL)3/RConn1 -- CB1/LConn1 -- Wind Turbine 1(GFL)2/RConn1 -- Wind Turbine 1(GFL)1/RConn1
  CB1/RConn1 -- Current and Voltage Sensor (Three-Phase)1/LConn1
